simulink model "mat3_PID_V1_2019b"  (R2019b)
settings: Solver=FixedStepAuto  StartTime=0.0  StopTime=8  RelTol=1e-3
libraries: arduinolib x4, simulink x2
settings Model: SILPILModeSetting=veronly  ExtModeTrigDuration=2  Creator=MU  LastModifiedBy=MU
settings DataIOCC: ReturnWorkspaceOutputs=off
settings OptimizationCC: EnhancedBackFolding=on  PassReuseOutputArgsAs=Individual arguments  ZeroExternalMemoryAtStartup=off  ZeroInternalMemoryAtStartup=off  MaxStackSize=64  OptimizeBlockOrder=speed  DifferentSizesBufferReuse=on  EfficientTunableParamExpr=on
settings DebuggingCC: ParameterTunabilityLossMsg=error
settings HardwareCC: ProdBitPerInt=16  ProdBitPerPointer=16  ProdBitPerSizeT=16  ProdBitPerPtrDiffT=16  ProdLargestAtomicFloat=None  ProdWordSize=8  ProdHWDeviceType=Atmel->AVR  UseEmbeddedCoderFeatures=off  UseSimulinkCoderFeatures=off
settings SFSimCC: MATLABDynamicMemAlloc=off
settings RTWCC: SystemTargetFile=ert.tlc  HardwareBoard=Arduino Mega 2560  TLCOptions=-aInlineSetEventsForThisBaseRateFcn=TLC_FALSE -aSuppressMultiTaskScheduler=TLC_FALSE -aRateBasedStepFcn=1  TemplateMakefile=ert_default_tmf  GenerateReport=on  Toolchain=Arduino AVR  BuildConfiguration=Faster Runs  IncludeHyperlinkInReport=on  LaunchReport=on  GenerateTraceInfo=on  GenerateTraceReport=on  GenerateTraceReportSl=on  GenerateTraceReportSf=on  GenerateTraceReportEml=on
settings CodeAppCC: ForceParamTrailComments=on  IgnoreCustomStorageClasses=off  OperatorAnnotations=on  SimulinkDataObjDesc=on  SFDataObjDesc=on  InsertBlockDesc=on
settings ERTTargetCC: SupportContinuousTime=on  SupportNonInlinedSFcns=on  SupportVariableSizeSignals=on  ExtModeStaticAllocSize=2048

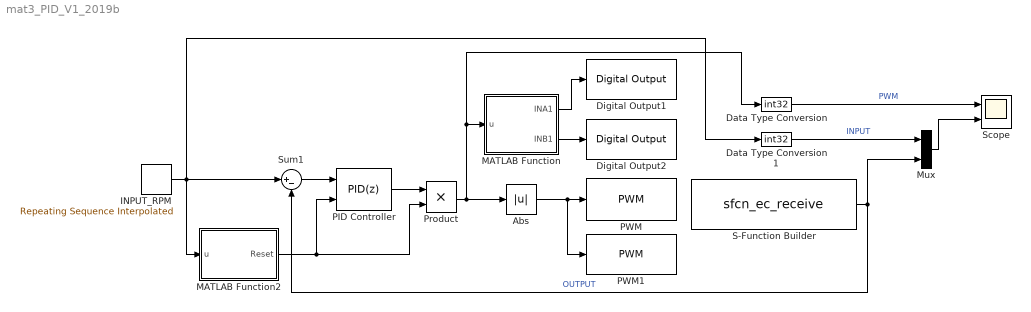
== system mat3_PID_V1_2019b ==
  Abs : Abs
  Data Type Conversion : DataTypeConversion  OutDataTypeStr=int32
  Data Type Conversion1 : DataTypeConversion  OutDataTypeStr=int32
  Digital Output1 : arduinolib/Digital Output  pinNumber=2  blockPlatform=arduino
  Digital Output2 : arduinolib/Digital Output  pinNumber=4  blockPlatform=arduino
  INPUT_RPM : simulink/Sources/Repeating Sequence Interpolated  OutValues=[0 0 30000 30000 -30000 -30000 -15000 -15000 2000 2000 15000 15000].'  TimeValues=[0 1 1.001 2 2.001 3 3.001 4 5 6 7 8].'  LookUpMeth=Interpolation-Use End Values  tsamp=0.0025  OutMin=[]  OutMax=[]  OutDataTypeStr=double  OutputDataTypeScalingMode=double  OutDataType=fixdt(0,8)  OutScaling=2^-10
  MATLAB Function : MATLAB Function  TreatAsAtomicUnit=on
  MATLAB Function2 : MATLAB Function  TreatAsAtomicUnit=on
  Mux : Mux  Inputs=2
  PID Controller : simulink/Continuous/PID Controller  Controller=PID  Form=Parallel  TimeDomain=Discrete-time  SampleTime=-1  IntegratorMethod=Forward Euler  FilterMethod=Forward Euler  ControllerParametersSource=internal  P=0.0165730931575491  I=0.464517742352602  D=0.0000693814314741502  UseFilter=on  N=109.47185061038  TunerSelectOption=Transfer Function Based (PID Tuner App)  InitialConditionSource=internal  InitialConditionForIntegrator=0  InitialConditionForFilter=0  DifferentiatorICPrevScaledInput=0  ExternalReset=either  TrackingMode=off  Kt=1  LimitOutput=on  UpperSaturationLimit=255  LowerSaturationLimit=-255  LinearizeAsGain=on  AntiWindupMode=none  Kb=1  POutMin=[]  POutMax=[]  IOutMin=[]  IOutMax=[]  DOutMin=[]  DOutMax=[]  NOutMin=[]  NOutMax=[]  SumOutMin=[]  SumOutMax=[]  SaturationOutMin=[]  SaturationOutMax=[]  PParamMin=[]  PParamMax=[]  IParamMin=[]  IParamMax=[]  DParamMin=[]  DParamMax=[]  NParamMin=[]  NParamMax=[]  KbParamMin=[]  KbParamMax=[]  KtParamMin=[]  KtParamMax=[]  KbOutMin=[]  KbOutMax=[]  KtOutMin=[]  KtOutMax=[]  IntegratorOutMin=[]  IntegratorOutMax=[]  FilterOutMin=[]  FilterOutMax=[]  SumI1OutMin=[]  SumI1OutMax=[]  SumI2OutMin=[]  SumI2OutMax=[]  SumI3OutMin=[]  SumI3OutMax=[]  SumI4OutMin=[]  SumI4OutMax=[]  SumDOutMin=[]  SumDOutMax=[]  DifferentiatorOutMin=[]  DifferentiatorOutMax=[]  FilterDiffOutCoefMin=[]  FilterDiffOutCoefMax=[]  ReciprocalOutMin=[]  ReciprocalOutMax=[]  SumDenOutMin=[]  SumDenOutMax=[]  SumNumOutMin=[]  SumNumOutMax=[]  DivideOutMin=[]  DivideOutMax=[]  IntegratorContinuousStateAttributes=''  IntegratorStateMustResolveToSignalObject=off  IntegratorRTWStateStorageClass=Auto  FilterContinuousStateAttributes=''  FilterStateMustResolveToSignalObject=off  FilterRTWStateStorageClass=Auto  ParallelPVariant=InternalParameters  IdealPVariant=Disabled  IVariant=InternalParameters  DVariant=InternalParameters  IntegratorVariant=Discrete  SatVariant=Enabled  AWVariant=Passthrough  PCopyVariant=Disabled  TRVariant=Disabled  FdbkBlocksVariant=Forward  IdealPFdbkVariant=Disabled  SatFdbkVariant=Disabled  DerivativeFilterVariant=ForwardEulerFilter  NVariant=InternalParameters  NCopyVariant=Disabled  FilterICVariant=InternalICsFilter  IntegratorICVariant=InternalICs  ExternalResetVariant=ExternalReset  TRSumVariant=Passthrough  SumFdbkVariant=Disabled  SumVariant=Sum_PID
  PWM : arduinolib/PWM  pinNumber=9  EnableInputFrequency=off  InitialFrequency=2000  InitialDutyCycle=0  NotificationType=None  blockPlatform=arduino
  PWM1 : arduinolib/PWM  pinNumber=13  EnableInputFrequency=off  InitialFrequency=2000  InitialDutyCycle=0  NotificationType=None  blockPlatform=arduino
  Product : Product
  S-Function Builder : S-Function  InitFcn=try, set_param(gcb,'FunctionName','sfcn_ec_receive'), end  FunctionName=sfcn_ec_receive  Parameters=uint8(19),uint8(31)  SFunctionModules=sfcn_ec_receive_wrapper  SFunctionDeploymentMode=off  EnableBusSupport=off  mask(S-Function Builder){}
      mask help: Simulink:masks:SFunctionBuilder_MD
      mask init:
      | val = [[.9  0.75 0.75 1 1 .9 .9 1]',[1 1 0.75 0.75 .9 .9 1 .9]'];try , sys = get_param(gcb,'SfunBuilderFcnName');if isempty(sys), sys = get_param(gcb,'FunctionName'); end,catch, sys = get_param(gcb,'FunctionName'); end
      settings: CopyFcn=set_param(gcbh,'LinkStatus','none')  PreSaveFcn=try, set_param(gcb,'FunctionName','sfcn_ec_receive'), end  OpenFcn=sfunctionwizard(gcbh)
      mask Display: plot(val(:,1),val(:,2)),disp(sys), port_label('output',1,'enc_rpm')
  Scope : Scope  NumInputPorts=2
  Sum1 : Sum  Inputs=|+-
  wires:
  MATLAB Function/2(INB1) -> Digital Output2/1
  Abs/1 -> PWM1/1, PWM/1
  Product/1 -> Data Type Conversion/1, MATLAB Function/1(u), Abs/1
  MATLAB Function/1(INA1) -> Digital Output1/1
  Data Type Conversion/1 -> Scope/1  "PWM"
  S-Function Builder/1 -> Mux/2, Sum1/2  "OUTPUT"
  Sum1/1 -> PID Controller/1
  INPUT_RPM/1 -> MATLAB Function2/1(u), Data Type Conversion1/1, Sum1/1
  Data Type Conversion1/1 -> Mux/1  "INPUT"
  Mux/1 -> Scope/2
  PID Controller/1 -> Product/1
  MATLAB Function2/1(Reset) -> PID Controller/2, Product/2

== matlab function mat3_PID_V1_2019b/MATLAB Function2 ==
  data: u input; Reset output
function Reset  = fcn(u)
 if(u==0) %STOP
    Reset = 0;
 else
    Reset = 1;
 end
end

== matlab function mat3_PID_V1_2019b/MATLAB Function ==
  data: u input; INA1 output; INB1 output
function [INA1,INB1] = fcn(u)
 if(u<0) %CCW
    INA1 = 0;
    INB1 = 1;
 elseif(u==0) %STOP
    INA1 = 0;
    INB1 = 0;
 else %CW
    INA1 = 1;
    INB1 = 0;
 end
end
